simulink model "carromasa"  (Simulink 7.9)
settings: Solver=ode3  StartTime=0.0  StopTime=20.0  RelTol=1e-3
values from neighbouring files (symbols this model uses):
  b = 0.1    [consCarroMasa.m]
  k = 10    [consCarroMasa.m]
  m = 1    [consCarroMasa.m]
undefined symbols (not defined in the file or in its folder): sigbuilder_block
libraries: simulink x1
settings Model: Creator=VLADIMIR  LastModifiedBy=USCO
settings DebuggingCC: MultiTaskCondExecSysMsg=warning  MultiTaskRateTransMsg=warning  FcnCallInpInsideContextMsg=Use local settings  StrictBusMsg=Warning
settings GRTTargetCC: CombineOutputUpdateFcns=off  GRTInterface=on

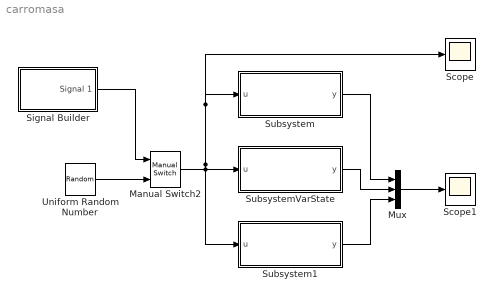
== system carromasa ==
  Manual Switch2 : simulink/Signal Routing/Manual Switch  sw=0  action=0  varsize=off
  Mux : Mux  Inputs=3
  Scope : Scope
      settings: SampleInput=on  SampleTime=0.1
  Scope1 : Scope
      settings: SampleInput=on  SampleTime=0.1
  Signal Builder : Subsystem  Tag=STV Subsys  LoadFcn=sigbuilder_block('load');  StartFcn=sigbuilder_block('start');  StopFcn=sigbuilder_block('stop');  ClipboardFcn=sigbuilder_block('clipboard');  mask(Sigbuilder block){}
      mask help: Sigbuilder GUI
      mask init:
      | if ~strcmp(get_param(bdroot(gcbh),'SimulationStatus'),'stopped') tuvar = sigbuilder_block('maskInit'); end
      settings: CopyFcn=sigbuilder_block('copy');  DeleteFcn=sigbuilder_block('delete');  ModelCloseFcn=sigbuilder_block('modelClose');  PreSaveFcn=sigbuilder_block('preSave');  PauseFcn=sigbuilder_block('pause')  ContinueFcn=sigbuilder_block('continue')  NameChangeFcn=sigbuilder_block('namechange');  OpenFcn=sigbuilder_block('open',[100.92 222.824 596.53 366.711 ]);  CloseFcn=sigbuilder_block('close');
      mask Display: plot(0,0,100,100,[10,10,40,40,10],[80,20,20,80,80],[40,10],[50,50], [40,27,10],[65,72,56],[40,25,25,10],[28,28,43,43]);
  Subsystem : Subsystem
  Subsystem1 : Subsystem
  SubsystemVarState : Subsystem
  Uniform Random Number : UniformRandomNumber  SampleTime=1
  wires:
  Mux/1 -> Scope1/1
  Subsystem/1(y) -> Mux/1
  SubsystemVarState/1(y) -> Mux/2
  Subsystem1/1(y) -> Mux/3
  Manual Switch2/1 -> SubsystemVarState/1(u), Subsystem1/1(u), Subsystem/1(u), Scope/1
  Signal Builder/1(Signal 1) -> Manual Switch2/1
  Uniform Random Number/1 -> Manual Switch2/2

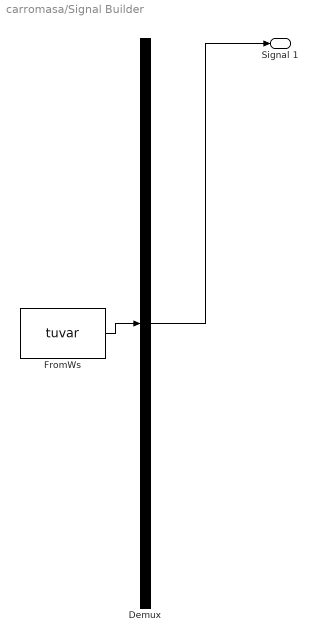
== system carromasa/Signal Builder ==
  Demux : Demux  Tag=STV Demux  Outputs=1
  FromWs : FromWorkspace  Tag=STV FromWs  VariableName=tuvar  SampleTime=0  SigBuilderData=DataTag0  VnvData=DataTag1
      SigBuilderData=|
      | common.afterFinalStr = 'Extrapolate'
      | common.sampleTime = 0
      | dataSet.timeRange = [0 10]
      | dataSet.name = 'Group 1'
      | sbobj.Groups.Name = 'Group 1'
      | sbobj.Groups.Signals.Name = 'Signal 1'
      | sbobj.Groups.Signals.XData = [0 4 4 5 5 10]
      | sbobj.Groups.Signals.YData = [0 0 0.5 0.5 0 0]
  Signal 1 : Outport  Tag=STV Outport
  wires:
  Demux/1 -> Signal 1/1
  FromWs/1 -> Demux/1

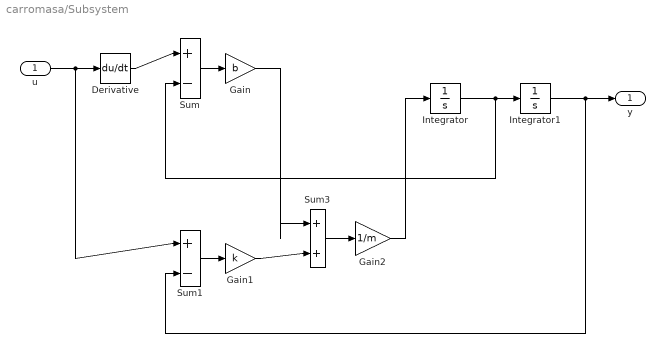
== system carromasa/Subsystem ==
  u : Inport
  Derivative : Derivative
  Gain : Gain  Gain=b
  Gain1 : Gain  Gain=k
  Gain2 : Gain  Gain=1/m
  Integrator : Integrator
  Integrator1 : Integrator
  Sum : Sum  Inputs=|+-
  Sum1 : Sum  Inputs=|+-
  Sum3 : Sum  Inputs=|++
  y : Outport
  wires:
  Integrator/1 -> Integrator1/1, Sum/2
  Integrator1/1 -> y/1, Sum1/2
  u/1 -> Derivative/1, Sum1/1
  Derivative/1 -> Sum/1
  Sum/1 -> Gain/1
  Sum1/1 -> Gain1/1
  Gain/1 -> Sum3/1
  Gain1/1 -> Sum3/2
  Sum3/1 -> Gain2/1
  Gain2/1 -> Integrator/1

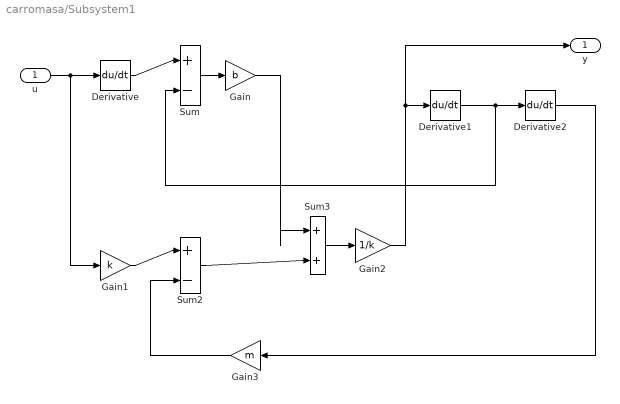
== system carromasa/Subsystem1 ==
  u : Inport
  Derivative : Derivative
  Derivative1 : Derivative
  Derivative2 : Derivative
  Gain : Gain  Gain=b
  Gain1 : Gain  Gain=k
  Gain2 : Gain  Gain=1/k
  Gain3 : Gain  Gain=m
  Sum : Sum  Inputs=|+-
  Sum2 : Sum  Inputs=|+-
  Sum3 : Sum  Inputs=|++
  y : Outport
  wires:
  Derivative1/1 -> Sum/2, Derivative2/1
  u/1 -> Derivative/1, Gain1/1
  Derivative/1 -> Sum/1
  Sum/1 -> Gain/1
  Gain/1 -> Sum3/1
  Sum3/1 -> Gain2/1
  Gain2/1 -> Derivative1/1, y/1
  Gain1/1 -> Sum2/1
  Derivative2/1 -> Gain3/1
  Gain3/1 -> Sum2/2
  Sum2/1 -> Sum3/2

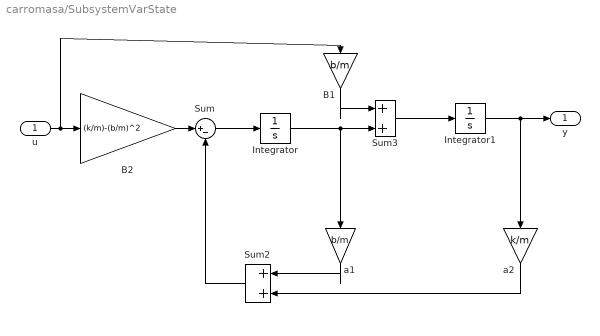
== system carromasa/SubsystemVarState ==
  u : Inport
  B1 : Gain  Gain=b/m
  B2 : Gain  Gain=(k/m)-(b/m)^2
  Integrator : Integrator
  Integrator1 : Integrator
  Sum : Sum  Inputs=|+-
  Sum2 : Sum  Inputs=|++
  Sum3 : Sum  Inputs=|++
  a1 : Gain  Gain=b/m
  a2 : Gain  Gain=k/m
  y : Outport
  wires:
  Integrator1/1 -> y/1, a2/1
  u/1 -> B2/1, B1/1
  B2/1 -> Sum/1
  Sum2/1 -> Sum/2
  Sum/1 -> Integrator/1
  Integrator/1 -> Sum3/2, a1/1
  a1/1 -> Sum2/1
  Sum3/1 -> Integrator1/1
  a2/1 -> Sum2/2
  B1/1 -> Sum3/1
